simulink model "MPPT_GSA"  (R2022a)
settings: Solver=VariableStepAuto  StartTime=0.0  StopTime=10.0  RelTol=1e-3
libraries: spsSeriesRLCBranchLib x4, spsCurrentMeasurementLib x1, spsDiodeLib x1, spsIGBTDiodeLib x1, spsPVArrayLib x1, spsPWMGeneratorDCDCLib x1, spsVoltageMeasurementLib x1, spspowerguiLib x1
settings Model: Creator=ASUS  LastModifiedBy=Thanh Quang
settings SolverCC: AlgebraicLoopSolver=LineSearch
settings DebuggingCC: UnconnectedInputMsg=warning  UnconnectedOutputMsg=warning  UnconnectedLineMsg=warning  SFMachineParentedDataDiag=warning
settings SFSimCC: CustomCodeUndefinedFunction=UseInterfaceOnly

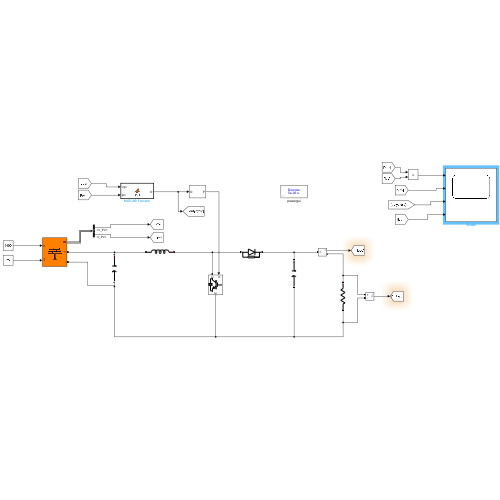
[thumbnail: Simulink's stored preview of the top-level diagram]
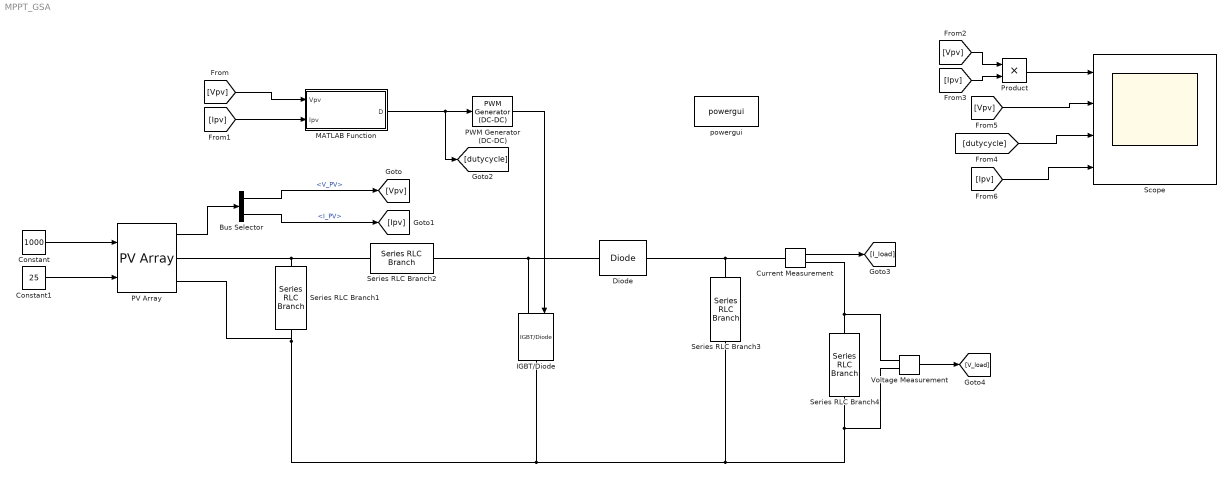
== system MPPT_GSA ==
  Bus Selector : BusSelector  OutputSignals=V_PV,I_PV
  Constant : Constant  Value=1000
  Constant1 : Constant  Value=25
  Current Measurement : spsCurrentMeasurementLib/Current Measurement  PhasorSimulation=off  OutputType=Complex  PSBequivalent=0
  Diode : spsDiodeLib/Diode  Ron=0.001  Lon=0  Vf=0.8  IC=0  UseSnubber=0  Rs=500  Cs=250e-9  Measurements=off
  IGBT/Diode : spsIGBTDiodeLib/IGBT//Diode  Ron=1e-3  Rs=1e5  Cs=inf  Measurements=off
  MATLAB Function : MATLAB Function  TreatAsAtomicUnit=on
  PV Array : spsPVArrayLib/PV Array  Npar=1  Nser=1  PlotType=array @ 25 deg.C & specified irradiances  S_vec="[ 1000  400 ]"  Temp_C_vec="[ 45 25  ]"  ModuleName=User-defined  PlotWhenSelected=off  Pm=248.977  Ncell=60  Voc=38.4  Isc=8.85  Vm=30.7  Im=8.11  beta_Voc_pc=-0.35599  alpha_Isc_pc=0.07  beta_Voc=-0.1367  alpha_Isc=0.006195  IL=8.8816  I0=2.622e-10  nI=1.0292  Rsh=104.8955  Rs=0.37421  RobustModel=off  RobustCellTemperature=313.3991  BAL=off  Tc=1e-6  Tfilter=5e-5
  PWM Generator (DC-DC) : spsPWMGeneratorDCDCLib/PWM Generator (DC-DC)  Fsw=5000  Ts=5e-6
  Product : Product
  Scope : Scope  NumInputPorts=4
  Series RLC Branch1 : spsSeriesRLCBranchLib/Series RLC Branch  LConnTagsString=__new0  RConnTagsString=__new0  BranchType=C  Resistance=1  Inductance=1e-3  SetiL0=off  InitialCurrent=0  Capacitance=100e-6  Setx0=off  InitialVoltage=0  Measurements=None
  Series RLC Branch2 : spsSeriesRLCBranchLib/Series RLC Branch  LConnTagsString=__new0  RConnTagsString=__new0  BranchType=L  Resistance=1  Inductance=1e-3  SetiL0=off  InitialCurrent=0  Capacitance=5e-3  Setx0=off  InitialVoltage=0  Measurements=None
  Series RLC Branch3 : spsSeriesRLCBranchLib/Series RLC Branch  LConnTagsString=__new0  RConnTagsString=__new0  BranchType=C  Resistance=1  Inductance=1e-3  SetiL0=off  InitialCurrent=0  Capacitance=12000e-6  Setx0=off  InitialVoltage=0  Measurements=None
  Series RLC Branch4 : spsSeriesRLCBranchLib/Series RLC Branch  LConnTagsString=__new0  RConnTagsString=__new0  BranchType=R  Resistance=10  Inductance=1e-3  SetiL0=off  InitialCurrent=0  Capacitance=12000e-6  Setx0=off  InitialVoltage=0  Measurements=None
  Voltage Measurement : spsVoltageMeasurementLib/Voltage Measurement  PhasorSimulation=off  OutputType=Complex  PSBequivalent=0
  powergui : spspowerguiLib/powergui  Priority=1  SimulationMode=Discrete  SampleTime=5e-6  frequency=60  Iterations=50  frequencyindice=0  Pbase=100e6  ErrMax=1e-4  UnitsV=kV  UnitsW=MW  buscounter=0  FunctionMessages=off  echomessages=off  EnableUseOfTLC=off  CurrentSourceSwitches=off  DisableSnubberDevices=off  DisableRonSwitches=off  DisableVfSwitches=off  DisplayEquations=off  AutomaticDiscreteSolvers=off  SolverType=Tustin/Backward Euler (TBE)  Interpol=off  ExternalGateDelay=off  methode=off  Ts=100  x0status=blocks  SPID=on  SwTol=0  HookPort=off  NonlinearTolerance=0  nMaxIteration=15  ContinueOnMaxIteration=off  RestoreLinks=warning  ResistiveCurrentMeasurement=off  Frange=[0:2:500]  Ylog=off  Xlog=on  ShowGrid=off  save=off  variable=ZData  structure=0  ZoomFFT=off  StartTime=0.0  cycles=1  DisplayStyle=1  fundamental=60  FreqAxis=off  MaxFrequency=1000  frequencyindicesteady=1  RmsSteady=1  display=off
  wires:
  PV Array/1 -> Bus Selector/1
  Constant/1 -> PV Array/1
  Constant1/1 -> PV Array/2
  Bus Selector/1 -> [Vpv]  "<V_PV>"
  Bus Selector/2 -> [Ipv]  "<I_PV>"
  [Vpv] -> MATLAB Function/1(Vpv)
  [Ipv] -> MATLAB Function/2(Ipv)
  MATLAB Function/1(D) -> [dutycycle], PWM Generator (DC-DC)/1
  PWM Generator (DC-DC)/1 -> IGBT/Diode/1
  [Vpv] -> Product/1
  [Ipv] -> Product/2
  Product/1 -> Scope/1
  Current Measurement/1 -> [I_load]
  Voltage Measurement/1 -> [V_load]
  [Vpv] -> Scope/2
  [dutycycle] -> Scope/3
  [Ipv] -> Scope/4
  connections:
  PV Array/RConn1 -- Series RLC Branch2/RConn1 -- Series RLC Branch1/LConn1
  Diode/LConn1 -- Series RLC Branch2/LConn1 -- IGBT/Diode/LConn1
  Series RLC Branch3/LConn1 -- Current Measurement/LConn1 -- Diode/RConn1
  Series RLC Branch4/RConn1 -- Voltage Measurement/LConn2 -- Series RLC Branch3/RConn1 -- PV Array/RConn2 -- Series RLC Branch1/RConn1 -- IGBT/Diode/RConn1
  Current Measurement/RConn1 -- Voltage Measurement/LConn1 -- Series RLC Branch4/LConn1

== matlab function MPPT_GSA/MATLAB Function ==
  data: Vpv input; D output; Ipv input
function D = GSA(Vpv,Ipv)
%%CHECKED%%
persistent u;%u-th particle
persistent dcurrent;%store current duty cycle
persistent pbest;%store local best dc for power
persistent force; %store force
persistent acceleration; %store acceleration
persistent mass; % mass
persistent q; %  strength of mass
persistent p; %  power for each particle
persistent p_current; %  power current for each particle
persistent p_min; %  power min for each particle
persistent worse;   %store best worse of each particle 
persistent dc; %store duty cycle ~ position 
persistent v;  %velocity
persistent counter; %delay iteration
persistent iteration;
persistent gbest;%store global best dc for power
%initialization
num_agency = 3;
max_iter = 500;
if(isempty(counter))
    counter = 0;
    dcurrent = 0.5; 
    gbest = 0.5;
    pbest = zeros(num_agency,1);
    worse = zeros(num_agency,1);
    v = zeros (num_agency,1);
    force = zeros(num_agency,1);
    mass = zeros(num_agency,1);
    q = zeros(num_agency,1);
    p = zeros(num_agency,1);
    p_current = zeros(num_agency,1);
    p_min=zeros(num_agency,1);
    p_min(1)= Vpv*Ipv;
    p_min(2)= Vpv*Ipv;
    p_min(3)= Vpv*Ipv;
    acceleration=zeros(num_agency,1);
    u = 0;
    dc = zeros (num_agency,1); 
    iteration = 1;
    
    %initialize position for each particle
    dc(1) = 0.2;
    dc(2) = 0.5;
    dc(3) = 0.8;
end

if(counter >=1 && counter < 100)
    D=dcurrent;
    counter= counter+1;
    return;
end

if(u>=1 && u<=num_agency)
    p_current(u) = Vpv*Ipv;
    if((Vpv*Ipv)>=p(u))
        p(u) = Vpv*Ipv;
        pbest(u)=dcurrent;
    end
    if(Vpv*Ipv < p_min(u))
        p_min(u) = Vpv*Ipv;
        worse(u) = dcurrent;
    end
end
u=u+1;
if(u== num_agency + 2)
    u=1;
end
if(u >= 1 && u <= num_agency)
    %Avoid over shooting
    if(iteration < max_iter)
        D=dc(u);
        dcurrent=D;
        counter=1;
    return;
    else
        D = dcurrent;
        return
    end
elseif(u==num_agency+1)
    iteration = iteration +1;
    [~,i]=max(p);
    gbest=pbest(i);
    D=gbest;
    dcurrent=D;
    counter=1;
     %Calculate strength of mass
    for i = 1:num_agency
     q(i) = (p_current(i) - worse(i))/(pbest(i)-worse(i));
    end
     %Calculate sum of strength of mass

     sum_strength_of_mass = q(1) + q(2) + q(3);
    
    %Calculate mass   
    for i = 1:num_agency
     mass(i) = q(i)/sum_strength_of_mass;
    
    end
    %Calculate force
    alpha = 20;
    G0 = 1;
    G = G0 * exp(-alpha*iteration/max_iter);
    %G = 6.67430 * 10^-13; %gravitational constant
    e = 2.2204*10^-16;
    force(1) = rand()*G*(mass(3)*mass(1)*(dc(3)-dc(1))/(Euclidian_distance(dc(3),dc(1))+e) + mass(2)*mass(1)*(dc(3)-dc(1))/(Euclidian_distance(dc(3),dc(1))+e));
    force(2) = rand()*G*(mass(3)*mass(2)*(dc(3)-dc(2))/(Euclidian_distance(dc(3),dc(2))+e) + mass(1)*mass(2)*(dc(1)-dc(2))/(Euclidian_distance(dc(1),dc(2))+e));
    force(3) = rand()*G*(mass(2)*mass(3)*(dc(2)-dc(3))/(Euclidian_distance(dc(2),dc(3))+e) + mass(1)*mass(3)*(dc(1)-dc(3))/(Euclidian_distance(dc(1),dc(3))+e));
    %Avoid over shooting
    if(iteration > max_iter)
        disp("should done")
        D=dcurrent;
        return;
    end
    %Calculate acceleration 
    for i = 1:num_agency
        acceleration(i) = force(i)/mass(i);
         disp(force(i))
    end
    
    for i=1:num_agency  
     v(i)=updatevelocity(v(i),acceleration(i));
     dc(i)=updateduty(dc(i),v(i));
     
    end  
    return;
    
else
    D=0.5
end
end
function d = Euclidian_distance(d1,d2)
    d = sqrt(d1^2+d2^2);
end
function vfinal=updatevelocity(velocity,acceleration)
    vfinal = rand()*velocity + acceleration;
end

function dfinal=updateduty(d,velocity)
dup=d+velocity;
if(dup>1)
    dfinal=1;
elseif(dup<0.1)
    dfinal=0,1;
else
    dfinal=dup;
end
end
